simulink model "StageFilterSimulation16thOrder"  (R2016b)
settings: Solver=FixedStepAuto  StartTime=0.0  StopTime=10/500  FixedStep=Ts  RelTol=1e-3
values from neighbouring files (symbols this model uses):
  A_in = floor(peak * 0.8)    [FilterDesign.m]
  A_noise = floor(peak * 0.1)    [FilterDesign.m]
  den = coeff(1:coeffdim(1),(coeffdim(2)/2 + 1):coeffdim(2))    [FilterDesign.m]
  f_in = 500    [FilterDesign.m]
  f_noise = 5e3    (= 5000)    [FilterDesign.m]
  num = coeff(1:coeffdim(1),1:(coeffdim(2)/2))    [FilterDesign.m]
  Ts = 1/fs    (= 1.024e-05)    [FilterDesign.m]
settings Model: Creator=alexis  LastModifiedBy=alexis
settings DebuggingCC: ParameterPrecisionLossMsg=none

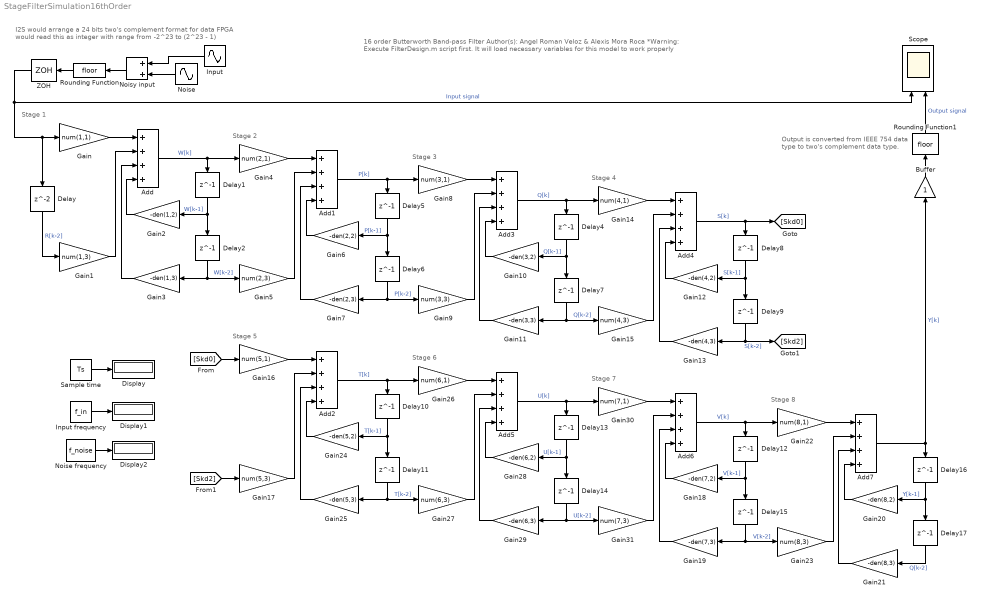
== system StageFilterSimulation16thOrder ==
  note: Output is converted from IEEE 754 data
      | type to two's complement data type.
  note: I2S would arrange a 24 bits two's complement format for data
      | FPGA would read this as integer with range from -2^23 to (2^23 - 1)
  note: 16 order Butterworth Band-pass Filter
      | Author(s): Angel Roman Veloz & Alexis Mora Roca
      | *Warning: Execute FilterDesign.m script first. It will load necessary variables for this model to work properly
  note: Stage 1
  note: Stage 2
  note: Stage 3
  note: Stage 4
  note: Stage 6
  note: Stage 7
  note: Stage 8
  note: Stage 5
  Add{,1..7} (8 alike) : Sum  Inputs=4
  Buffer : Gain
  Delay : Delay
  Delay{1..2,4..17} (16 alike) : Delay  DelayLength=1
  Display : Display
  Display1 : Display
  Display2 : Display
  Gain : Gain  Gain=num(1,1)
  Gain1 : Gain  Gain=num(1,3)
  Gain10 : Gain  Gain=-den(3,2)
  Gain11 : Gain  Gain=-den(3,3)
  Gain12 : Gain  Gain=-den(4,2)
  Gain13 : Gain  Gain=-den(4,3)
  Gain14 : Gain  Gain=num(4,1)
  Gain15 : Gain  Gain=num(4,3)
  Gain16 : Gain  Gain=num(5,1)
  Gain17 : Gain  Gain=num(5,3)
  Gain18 : Gain  Gain=-den(7,2)
  Gain19 : Gain  Gain=-den(7,3)
  Gain2 : Gain  Gain=-den(1,2)
  Gain20 : Gain  Gain=-den(8,2)
  Gain21 : Gain  Gain=-den(8,3)
  Gain22 : Gain  Gain=num(8,1)
  Gain23 : Gain  Gain=num(8,3)
  Gain24 : Gain  Gain=-den(5,2)
  Gain25 : Gain  Gain=-den(5,3)
  Gain26 : Gain  Gain=num(6,1)
  Gain27 : Gain  Gain=num(6,3)
  Gain28 : Gain  Gain=-den(6,2)
  Gain29 : Gain  Gain=-den(6,3)
  Gain3 : Gain  Gain=-den(1,3)
  Gain30 : Gain  Gain=num(7,1)
  Gain31 : Gain  Gain=num(7,3)
  Gain4 : Gain  Gain=num(2,1)
  Gain5 : Gain  Gain=num(2,3)
  Gain6 : Gain  Gain=-den(2,2)
  Gain7 : Gain  Gain=-den(2,3)
  Gain8 : Gain  Gain=num(3,1)
  Gain9 : Gain  Gain=num(3,3)
  Input : Sin  Amplitude=A_in  Frequency=2*pi*f_in  SampleTime=0
  Input frequency : Constant  Value=f_in
  Noise : Sin  Amplitude=A_noise  Frequency=2*pi*f_noise  SampleTime=0
  Noise frequency : Constant  Value=f_noise
  Noisy input : Sum
  Rounding Function : Rounding
  Rounding Function1 : Rounding
  Sample time : Constant  Value=Ts
  Scope : Scope  NumInputPorts=2
  ZOH : ZeroOrderHold  SampleTime=-1
  wires:
  Delay/1 -> Gain1/1  "R[k-2]"
  Gain/1 -> Add/1
  Gain1/1 -> Add/2
  Delay1/1 -> Gain2/1, Delay2/1  "W[k-1]"
  Delay2/1 -> Gain5/1, Gain3/1  "W[k-2]"
  Gain2/1 -> Add/4
  Gain3/1 -> Add/3
  Add/1 -> Gain4/1, Delay1/1  "W[k]"
  Gain4/1 -> Add1/1
  Gain5/1 -> Add1/2
  Delay5/1 -> Gain6/1, Delay6/1  "P[k-1]"
  Delay6/1 -> Gain9/1, Gain7/1  "P[k-2]"
  Gain6/1 -> Add1/4
  Gain7/1 -> Add1/3
  Add1/1 -> Gain8/1, Delay5/1  "P[k]"
  Gain8/1 -> Add3/1
  Gain9/1 -> Add3/2
  Delay4/1 -> Gain10/1, Delay7/1  "Q[k-1]"
  Delay7/1 -> Gain15/1, Gain11/1  "Q[k-2]"
  Gain10/1 -> Add3/4
  Gain11/1 -> Add3/3
  Add3/1 -> Gain14/1, Delay4/1  "Q[k]"
  Gain14/1 -> Add4/1
  Gain15/1 -> Add4/2
  Delay8/1 -> Gain12/1, Delay9/1  "S[k-1]"
  Delay9/1 -> Gain13/1, [Skd2]  "S[k-2]"
  Gain12/1 -> Add4/4
  Gain13/1 -> Add4/3
  Add4/1 -> [Skd0], Delay8/1  "S[k]"
  ZOH/1 -> Scope/1, Delay/1, Gain/1  "Input signal"
  Gain16/1 -> Add2/1
  Gain17/1 -> Add2/2
  Delay10/1 -> Gain24/1, Delay11/1  "T[k-1]"
  Delay11/1 -> Gain27/1, Gain25/1  "T[k-2]"
  Gain24/1 -> Add2/4
  Gain25/1 -> Add2/3
  Add2/1 -> Gain26/1, Delay10/1  "T[k]"
  Gain26/1 -> Add5/1
  Gain27/1 -> Add5/2
  Delay13/1 -> Gain28/1, Delay14/1  "U[k-1]"
  Delay14/1 -> Gain31/1, Gain29/1  "U[k-2]"
  Gain28/1 -> Add5/4
  Gain29/1 -> Add5/3
  Add5/1 -> Gain30/1, Delay13/1  "U[k]"
  Gain30/1 -> Add6/1
  Gain31/1 -> Add6/2
  Delay12/1 -> Gain18/1, Delay15/1  "V[k-1]"
  Delay15/1 -> Gain23/1, Gain19/1  "V[k-2]"
  Gain18/1 -> Add6/4
  Gain19/1 -> Add6/3
  Add6/1 -> Gain22/1, Delay12/1  "V[k]"
  Gain22/1 -> Add7/1
  Gain23/1 -> Add7/2
  Delay16/1 -> Gain20/1, Delay17/1  "Y[k-1]"
  Delay17/1 -> Gain21/1  "Q[k-2]"
  Gain20/1 -> Add7/4
  Gain21/1 -> Add7/3
  Add7/1 -> Delay16/1, Buffer/1  "Y[k]"
  [Skd0] -> Gain16/1
  [Skd2] -> Gain17/1
  Noise/1 -> Noisy input/2
  Input/1 -> Noisy input/1
  Sample time/1 -> Display/1
  Input frequency/1 -> Display1/1
  Noise frequency/1 -> Display2/1
  Rounding Function/1 -> ZOH/1
  Noisy input/1 -> Rounding Function/1
  Buffer/1 -> Rounding Function1/1
  Rounding Function1/1 -> Scope/2  "Output signal"
